simulink model "mls_driver_nasz_2015a_LQR"  (R2015a)
settings: Solver=ode5  SolverMode=SingleTasking  StartTime=0.0  StopTime=inf  FixedStep=0.001  RelTol=1e-3  AbsTol=1e-6
InitFcn:
  | load ml_sensor
values from neighbouring files (symbols this model uses):
  A_LC = A_obs - L*C_obs    [linearize_model.m]
  B_obs = B(1:3)    [linearize_model.m]
  i_ep = op.States(3).x    [linearize_model.m]
  Kc = lqr(A,B,Q,R)    [linearize_model.m]
  L = transpose(place(transpose(A_obs),C_obs.',eig_val))    [linearize_model.m]
  u_ep = op.Inputs(1).u    [linearize_model.m]
  z_ep = op.States(1).x    [linearize_model.m]
undefined symbols (not defined in the file): RTDAC4PCIBaseAddress
libraries: simulink x1
settings Model: SimulationMode=external  CovHtmlReporting=off  CovSFcnEnable=off  ExtModeEnableFloating=off  ExtModeTrigDuration=120000  ExtModeTrigDirection=either  ExtModeArchiveFileName=exp01.mat  ExtModeArchiveDirName=h:\temp  ExtModeWriteAllDataToWs=on  Creator=Adam Pilat  LastModifiedBy=Student
settings DataIOCC: ExternalInput=[]  InitialState=[]  LimitDataPoints=off  MaxDataPoints=5000  SignalLoggingSaveFormat=ModelDataLogs  SaveOutput=off  SaveTime=off  SignalLoggingName=sigsOut
settings OptimizationCC: BooleanDataType=off  ExpressionDepthLimit=2147483647  InitFltsAndDblsToZero=on
settings DebuggingCC: SaveWithParameterizedLinksMsg=none  UnderspecifiedInitializationDetection=Classic  MergeDetectMultiDrivingBlocksExec=none  SignalResolutionControl=TryResolveAllWithWarning  MultiTaskDSMMsg=warning  MultiTaskCondExecSysMsg=none  IntegerOverflowMsg=none  FcnCallInpInsideContextMsg=EnableAllAsWarning  StateNameClashWarn=warning  IntegerSaturationMsg=none
settings HardwareCC: ProdBitPerLong=64  ProdBitPerPointer=64  ProdIntDivRoundTo=Zero  ProdEndianess=LittleEndian  ProdWordSize=64  ProdHWDeviceType=Intel->x86-64  TargetBitPerLong=64  TargetBitPerPointer=64  TargetIntDivRoundTo=Zero  TargetEndianess=LittleEndian  TargetWordSize=64  TargetHWDeviceType=Intel->x86-64
settings RTWCC: SystemTargetFile=rtwin.tlc  TemplateMakefile=rtwin.tmf  Description=Real-Time Windows Target
settings TargetCC: TargetFcnLib=ansi_tfl_tmw.mat  TargetPreCompLibLocation=C:\Program Files\MATLAB\R2015aSP1\toolbox\sldrt\lib\win64  ModelReferenceCompliant=off  CompOptLevelCompliant=off  GeneratePreprocessorConditionals=Use local settings

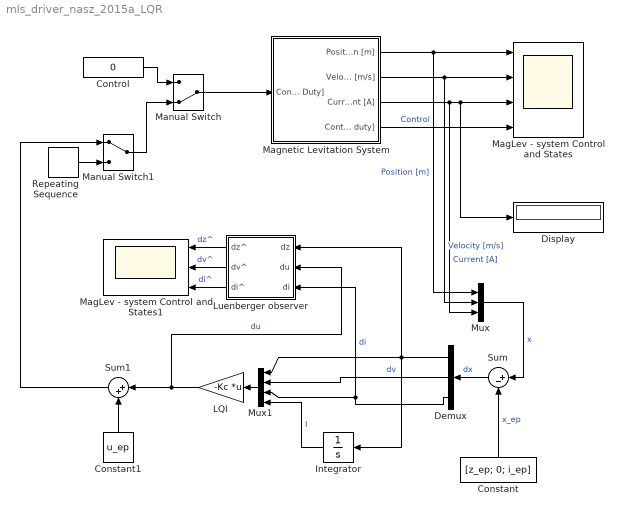
== system mls_driver_nasz_2015a_LQR ==
  Constant : Constant  Value=[z_ep; 0; i_ep]
  Constant1 : Constant  Value=u_ep
  Control : Constant  Value=0
  Demux : Demux  Outputs=3
  Display : Display
  Integrator : Integrator
  LQI : Gain  Gain=-Kc  Multiplication=Matrix(K*u) (u vector)
  Luenberger observer : Subsystem
  MagLev - system Control and States : Scope  NumInputPorts=4
      settings: TimeRange=10.1  YMin=0.009875~-0.04~0.9~0  YMax=0.010175~0.04~1.125~1  SaveName=MLExpData  MaxDataPoints=10000
  MagLev - system Control and States1 : Scope  NumInputPorts=3
      settings: TimeRange=10.1  YMin=-410.6~-905.25~-3320  YMax=-408.7~-900.5~-3304  SaveName=MLExpData1  MaxDataPoints=10000
  Magnetic Levitation System : Subsystem  mask(Magnetic Levitation 1 - System){BA=RTDAC4PCIBaseAddress, T0=0.001}
      mask prompts: BA "Base Address (dec):"; T0 "Sampling period [s]:"
      mask help:
      | MagLev1 - System connection for the real-time operating mode
      | (c) InTeCo 2005
      mask Display: image(imread('MagLev1.tif'))
  Manual Switch : ManualSwitch  CurrentSetting=0
  Manual Switch1 : ManualSwitch
  Mux : Mux  Inputs=3
  Mux1 : Mux
  Repeating Sequence : simulink/Sources/Repeating Sequence  rep_seq_t=[0 1 10]  rep_seq_y=[0 1 1]
  Sum : Sum  Inputs=|+-
  Sum1 : Sum  Inputs=|++
  wires:
  Magnetic Levitation System/1(Position [m]) -> Mux/1, MagLev - system Control and States/1  "Position [m]"
  Magnetic Levitation System/2(Velocity [m/s]) -> Mux/2, MagLev - system Control and States/2  "Velocity [m/s]"
  Magnetic Levitation System/3(Current [A]) -> Mux/3, Display/1, MagLev - system Control and States/3  "Current [A]"
  Magnetic Levitation System/4(Control [PWM duty]) -> MagLev - system Control and States/4  "Control"
  Manual Switch/1 -> Magnetic Levitation System/1(Control [PWM Duty])
  Control/1 -> Manual Switch/1
  Sum1/1 -> Manual Switch1/1
  Mux/1 -> Sum/1  "x"
  Constant/1 -> Sum/2  "x_ep"
  Constant1/1 -> Sum1/2
  LQI/1 -> Luenberger observer/2(du), Sum1/1  "du"
  Repeating Sequence/1 -> Manual Switch1/2
  Manual Switch1/1 -> Manual Switch/2
  Sum/1 -> Demux/1  "dx"
  Demux/1 -> Mux1/1, Luenberger observer/1(dz), Integrator/1
  Mux1/1 -> LQI/1
  Integrator/1 -> Mux1/4  "I"
  Demux/3 -> Mux1/3, Luenberger observer/3(di)  "di"
  Demux/2 -> Mux1/2  "dv"
  Luenberger observer/1(dz^) -> MagLev - system Control and States1/1  "dz^"
  Luenberger observer/2(dv^) -> MagLev - system Control and States1/2  "dv^"
  Luenberger observer/3(di^) -> MagLev - system Control and States1/3  "di^"

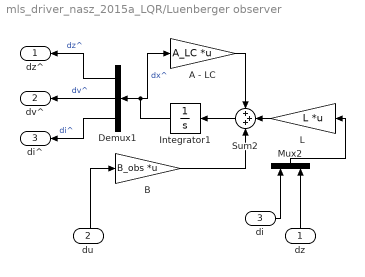
== system mls_driver_nasz_2015a_LQR/Luenberger observer ==
  dz : Inport
  du : Inport  Port=2
  di : Inport  Port=3
  A - LC : Gain  Gain=A_LC  Multiplication=Matrix(K*u) (u vector)
  B : Gain  Gain=B_obs  Multiplication=Matrix(K*u) (u vector)
  Demux1 : Demux  Outputs=3
  Integrator1 : Integrator
  L : Gain  Gain=L  Multiplication=Matrix(K*u) (u vector)
  Mux2 : Mux  Inputs=2
  Sum2 : Sum  Inputs=+++
  dz^ : Outport
  dv^ : Outport  Port=2
  di^ : Outport  Port=3
  wires:
  di/1 -> Mux2/1
  du/1 -> B/1
  dz/1 -> Mux2/2
  L/1 -> Sum2/2
  Sum2/1 -> Integrator1/1
  B/1 -> Sum2/3
  Mux2/1 -> L/1
  Integrator1/1 -> Demux1/1, A - LC/1  "dx^"
  A - LC/1 -> Sum2/1
  Demux1/1 -> dz^/1  "dz^"
  Demux1/2 -> dv^/1  "dv^"
  Demux1/3 -> di^/1  "di^"

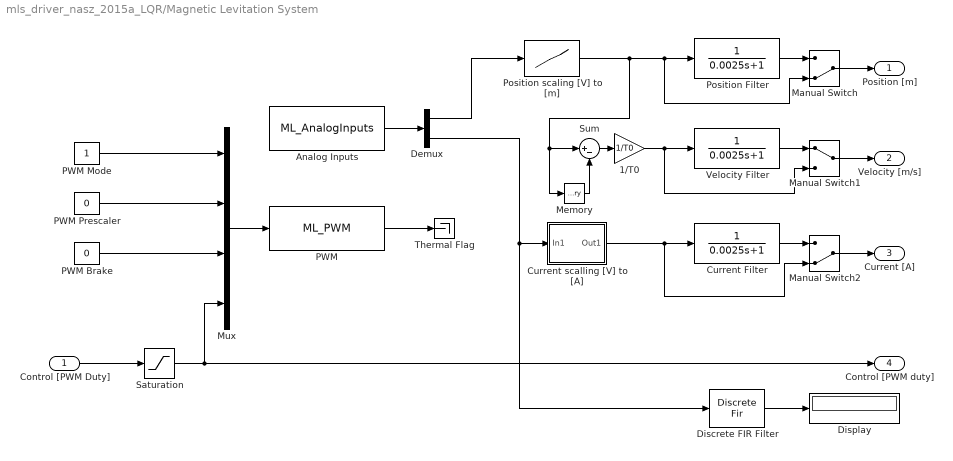
== system mls_driver_nasz_2015a_LQR/Magnetic Levitation System ==
  Control [PWM Duty] : Inport
  1/T0 : Gain  Gain=1/T0  SaturateOnIntegerOverflow=on  OutDataTypeStr=Inherit: Same as input  ParamDataTypeStr=Inherit: Same as input
  Analog Inputs : S-Function  FunctionName=ML_AnalogInputs  Parameters=BA, [4 2], [1 1], T0
  Current Filter : TransferFcn  Denominator=[0.0025 1]
  Current scalling [V] to [A] : Subsystem
      mask Display: plot([0    0.5000    1.0000    1.5000    2.0000    2.5000], [-0.0317    0.4951    1.0302    1.5738    2.1258    2.6863]);
  Demux : Demux  Outputs=2
  Discrete FIR Filter : DiscreteFir  Coefficients=ones(1,1000)/1000
  Display : Display
  Manual Switch : ManualSwitch  CurrentSetting=0
  Manual Switch1 : ManualSwitch
  Manual Switch2 : ManualSwitch  CurrentSetting=0
  Memory : Memory
  Mux : Mux
  PWM : S-Function  FunctionName=ML_PWM  Parameters=BA, T0
  PWM Brake : Constant  Value=0
  PWM Mode : Constant
  PWM Prescaler : Constant  Value=0
  Position Filter : TransferFcn  Denominator=[0.0025 1]
  Position scaling [V] to [m] : Lookup  InputValues=SensorData.Sensor_V(end:-1:1)  Table=SensorData.Distance_m(end:-1:1)  SaturateOnIntegerOverflow=on
  Saturation : Saturate  UpperLimit=1  LowerLimit=0
  Sum : Sum  Inputs=|+-  SaturateOnIntegerOverflow=on  InputSameDT=on  OutDataTypeStr=Inherit: Same as first input
  Thermal Flag : Terminator
  Velocity Filter : TransferFcn  Denominator=[0.0025 1]
  Position [m] : Outport
  Velocity [m/s] : Outport  Port=2
  Current [A] : Outport  Port=3
  Control [PWM duty] : Outport  Port=4
  wires:
  Manual Switch1/1 -> Velocity [m/s]/1
  Current Filter/1 -> Manual Switch2/1
  Velocity Filter/1 -> Manual Switch1/1
  Position Filter/1 -> Manual Switch/1
  Demux/1 -> Position scaling [V] to [m]/1
  Demux/2 -> Discrete FIR Filter/1, Current scalling [V] to [A]/1(In1)
  Current scalling [V] to [A]/1(Out1) -> Manual Switch2/2, Current Filter/1
  1/T0/1 -> Manual Switch1/2, Velocity Filter/1
  Sum/1 -> 1/T0/1
  Memory/1 -> Sum/2
  Analog Inputs/1 -> Demux/1
  Mux/1 -> PWM/1
  PWM Prescaler/1 -> Mux/2
  PWM Mode/1 -> Mux/1
  PWM/1 -> Thermal Flag/1
  Saturation/1 -> Mux/4, Control [PWM duty]/1
  Control [PWM Duty]/1 -> Saturation/1
  Manual Switch2/1 -> Current [A]/1
  PWM Brake/1 -> Mux/3
  Position scaling [V] to [m]/1 -> Manual Switch/2, Position Filter/1, Memory/1, Sum/1
  Manual Switch/1 -> Position [m]/1
  Discrete FIR Filter/1 -> Display/1

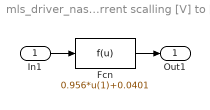
== system mls_driver_nasz_2015a_LQR/Magnetic Levitation System/Current scalling [V] to [A] ==
  In1 : Inport
  Fcn : Fcn  Expr=0.956*u(1)+0.0401
  Out1 : Outport
  wires:
  In1/1 -> Fcn/1
  Fcn/1 -> Out1/1
